simulink model "ALL_JP360_DBW_V6_5_1103"  (R2022a)
settings: Solver=FixedStepAuto  StartTime=0.0  StopTime=inf  FixedStep=0.01  RelTol=1e-3  EnableMultiTasking=on
model workspace (MAT data in the model file):
  g = 9.8
undefined symbols (not defined in the file or in its folder): canChannel, delta_v_p, IPM_Line_C0, IPM_Line_C1, IPM_Line_C2, IPM_Line_C3, M, M_p, MRR_ObjDistX, MRR_ObjDistY, MRR_ObjFusionCamID, MRR_ObjFusionSig, MRR_ObjID, MRR_ObjRelVelX, MRR_ObjRelVelY, MRR_ObjType, MRR_ObjUpdFlg, none, obj_vaild, untracktime, V, videoinput
libraries: canfdmsglib x230, canfdlib x76, slpidlib x24, simulink x18, dspstat3 x14, ctrlSharedLib x1, simulink_extras x1, imaqlib x1, realtime_pacer_lib x1, dspvision x1, visionsinks x1
(part 13 of 55)

== system ALL_JP360_DBW_V6_5_1103/MsgFromCAN/CCAN_GW_MsgFromCAN/CCAN_GW_ESP_Advanced_0x234 ==
  CCAN_GW_ESP_Advanced_0x234FromInData : Inport  OutDataTypeStr=Bus:CAN_FD_MESSAGE_BUS
  Bus Creator : BusCreator  Inputs=24  OutDataTypeStr=Bus:CCAN_GW_ESP_Advanced_0x234  NonVirtualBus=on
  CAN FD Unpack : canfdmsglib/CAN FD Unpack  CANdbFile=HiFire_JPT360_CCAN_Matrix_CAN_V1.72_VP_ADCU.dbc  MsgList=(none)  MsgName=ESP_Advanced_0x234  ProtocolMode=CAN FD  MsgIDType=Standard (11-bit identifier)  MsgIdentifier=564  MsgLength=8  SignalInfo={'Checksum_0x234','56','8','BE','unsigned','Standard','0','1','0','0','255';'ESP_ABAactive','22','1','BE','unsigned','Standard','0','1','0','0','1';'ESP_ABAavailable','21','1','BE','unsigned','Standard','0','1','0','0','1';'ESP_AEBdecActive','18','1','BE','unsigned','Standard','0','1','0','0','1';'ESP_AEBdecAvailable','17','1','BE','unsigned','Standard','0','1','0','0','1';'ESP_AWBactive','26','1','BE','unsigned','Standard','0','1','0','0','1';'ESP_AWBavailable','25','1','BE','unsigned','Standard','0','1','0','0','1';'ESP_BrkFricTqTotAtWhl','40','14','BE','unsigned','Standard','0','1','0','0','10230';'ESP_BrkFricTqTotAtWhlvaild','16','1','BE','unsigned','Standard','0','1','0','0','1';'ESP_CDDActive','8','1','BE','unsigned','Standard','0','1','0','0','1';'ESP_CDDAvailable','23','1','BE','unsigned','Standard','0','1','0','0','1';'ESP_CDD_APAactive','9','1','BE','unsigned','Standard','0','1','0','0','1';'ESP_CDDerror','39','1','BE','unsigned','Standard','0','1','0','0','1';'ESP_DTCactive','24','1','BE','unsigned','Standard','0','1','0','0','1';'ESP_EBDActive','1','1','BE','unsigned','Standard','0','1','0','0','1';'ESP_ECDTempOff','14','1','BE','unsigned','Standard','0','1','0','0','1';'ESP_HBBActive','54','1','BE','unsigned','Standard','0','1','0','0','1';'ESP_NoBrakeForce','15','1','BE','unsigned','Standard','0','1','0','0','1';'ESP_PrefillActive','20','1','BE','unsigned','Standard','0','1','0','0','1';'ESP_PrefillAvailable','19','1','BE','unsigned','Standard','0','1','0','0','1';'ESP_VAMActive','55','1','BE','unsigned','Standard','0','1','0','0','1';'ESP_VDCActive','0','1','BE','unsigned','Standard','0','1','0','0','1';'ESP_VLCerror','38','1','BE','unsigned','Standard','0','1','0','0','1';'RollingCounter_0x234','48','4','BE','unsigned','Standard','0','1','0','0','15'}  IDPort=off  TimestampPort=off  ErrorPort=off  RemotePort=off  LengthPort=off  StatusPort=off  BRSPort=off  ESIPort=off  DLCPort=off  ApplyMinMax=off
      settings: SourceProductBaseCode=XP,ME,VN  DataFormat=CANdb specified signals
  Data Type Conversion1 : DataTypeConversion  OutDataTypeStr=uint8  SaturateOnIntegerOverflow=off  RndMeth=Floor
  Data Type Conversion{2..7,9..23} (21 alike) : DataTypeConversion  OutDataTypeStr=boolean  SaturateOnIntegerOverflow=off  RndMeth=Floor
  Data Type Conversion24 : DataTypeConversion  OutDataTypeStr=int8  SaturateOnIntegerOverflow=off  RndMeth=Floor
  Data Type Conversion8 : DataTypeConversion  OutDataTypeStr=int16  SaturateOnIntegerOverflow=off  RndMeth=Floor
  CCAN_GW_ESP_Advanced_0x234FromOutData : Outport  OutDataTypeStr=Bus:CCAN_GW_ESP_Advanced_0x234
  wires:
  CAN FD Unpack/1 -> Data Type Conversion1/1
  CAN FD Unpack/2 -> Data Type Conversion2/1
  CAN FD Unpack/3 -> Data Type Conversion3/1
  CAN FD Unpack/4 -> Data Type Conversion4/1
  CAN FD Unpack/5 -> Data Type Conversion5/1
  CAN FD Unpack/6 -> Data Type Conversion6/1
  CAN FD Unpack/7 -> Data Type Conversion7/1
  CAN FD Unpack/8 -> Data Type Conversion8/1
  CAN FD Unpack/9 -> Data Type Conversion9/1
  CAN FD Unpack/10 -> Data Type Conversion10/1
  CAN FD Unpack/11 -> Data Type Conversion11/1
  CAN FD Unpack/12 -> Data Type Conversion12/1
  CAN FD Unpack/13 -> Data Type Conversion13/1
  CAN FD Unpack/14 -> Data Type Conversion14/1
  CAN FD Unpack/15 -> Data Type Conversion15/1
  CAN FD Unpack/16 -> Data Type Conversion16/1
  CAN FD Unpack/17 -> Data Type Conversion17/1
  CAN FD Unpack/18 -> Data Type Conversion18/1
  CAN FD Unpack/19 -> Data Type Conversion19/1
  CAN FD Unpack/20 -> Data Type Conversion20/1
  CAN FD Unpack/21 -> Data Type Conversion21/1
  CAN FD Unpack/22 -> Data Type Conversion22/1
  CAN FD Unpack/23 -> Data Type Conversion23/1
  CAN FD Unpack/24 -> Data Type Conversion24/1
  Data Type Conversion1/1 -> Bus Creator/1  "Checksum_0x234"
  Data Type Conversion2/1 -> Bus Creator/2  "ESP_ABAactive"
  Data Type Conversion3/1 -> Bus Creator/3  "ESP_ABAavailable"
  Data Type Conversion4/1 -> Bus Creator/4  "ESP_AEBdecActive"
  Data Type Conversion5/1 -> Bus Creator/5  "ESP_AEBdecAvailable"
  Data Type Conversion6/1 -> Bus Creator/6  "ESP_AWBactive"
  Data Type Conversion7/1 -> Bus Creator/7  "ESP_AWBavailable"
  Data Type Conversion8/1 -> Bus Creator/8  "ESP_BrkFricTqTotAtWhl"
  Data Type Conversion9/1 -> Bus Creator/9  "ESP_BrkFricTqTotAtWhlvaild"
  Data Type Conversion10/1 -> Bus Creator/10  "ESP_CDDActive"
  Data Type Conversion11/1 -> Bus Creator/11  "ESP_CDDAvailable"
  Data Type Conversion12/1 -> Bus Creator/12  "ESP_CDD_APAactive"
  Data Type Conversion13/1 -> Bus Creator/13  "ESP_CDDerror"
  Data Type Conversion14/1 -> Bus Creator/14  "ESP_DTCactive"
  Data Type Conversion15/1 -> Bus Creator/15  "ESP_EBDActive"
  Data Type Conversion16/1 -> Bus Creator/16  "ESP_ECDTempOff"
  Data Type Conversion17/1 -> Bus Creator/17  "ESP_HBBActive"
  Data Type Conversion18/1 -> Bus Creator/18  "ESP_NoBrakeForce"
  Data Type Conversion19/1 -> Bus Creator/19  "ESP_PrefillActive"
  Data Type Conversion20/1 -> Bus Creator/20  "ESP_PrefillAvailable"
  Data Type Conversion21/1 -> Bus Creator/21  "ESP_VAMActive"
  Data Type Conversion22/1 -> Bus Creator/22  "ESP_VDCActive"
  Data Type Conversion23/1 -> Bus Creator/23  "ESP_VLCerror"
  Data Type Conversion24/1 -> Bus Creator/24  "RollingCounter_0x234"
  Bus Creator/1 -> CCAN_GW_ESP_Advanced_0x234FromOutData/1  "CCAN_GW_ESP_Advanced_0x234FromOutData"
  CCAN_GW_ESP_Advanced_0x234FromInData/1 -> CAN FD Unpack/1  "CCAN_GW_ESP_Advanced_0x234FromInData"

== system ALL_JP360_DBW_V6_5_1103/MsgFromCAN/CCAN_GW_MsgFromCAN/CCAN_GW_ESP_AxAy_0x242 ==
  CCAN_GW_ESP_AxAy_0x242FromInData : Inport  OutDataTypeStr=Bus:CAN_FD_MESSAGE_BUS
  Bus Creator : BusCreator  Inputs=8  OutDataTypeStr=Bus:CCAN_GW_ESP_AxAy_0x242  NonVirtualBus=on
  CAN FD Unpack : canfdmsglib/CAN FD Unpack  CANdbFile=HiFire_JPT360_CCAN_Matrix_CAN_V1.72_VP_ADCU.dbc  MsgList=(none)  MsgName=ESP_AxAy_0x242  ProtocolMode=CAN FD  MsgIDType=Standard (11-bit identifier)  MsgIdentifier=578  MsgLength=8  SignalInfo={'Checksum_0x242','56','8','BE','unsigned','Standard','0','1','0','0','255';'ESP_Alat','16','12','BE','unsigned','Standard','0','0.027127','-21.5931','-21.5931','21.5931';'ESP_AlatStatus','54','1','BE','unsigned','Standard','0','1','0','0','1';'ESP_Algt','12','12','BE','unsigned','Standard','0','0.027127','-21.5931','-21.5931','21.5931';'ESP_AlgtStatus','55','1','BE','unsigned','Standard','0','1','0','0','1';'ESP_YawRate','36','12','BE','unsigned','Standard','0','0.001745','-2.0942','-2.0942','5.0498';'ESP_YawRateStatus','53','1','BE','unsigned','Standard','0','1','0','0','1';'RollingCounter_0x242','48','4','BE','unsigned','Standard','0','1','0','0','15'}  IDPort=off  TimestampPort=off  ErrorPort=off  RemotePort=off  LengthPort=off  StatusPort=off  BRSPort=off  ESIPort=off  DLCPort=off  ApplyMinMax=off
      settings: SourceProductBaseCode=XP,ME,VN  DataFormat=CANdb specified signals
  Data Type Conversion1 : DataTypeConversion  OutDataTypeStr=uint8  SaturateOnIntegerOverflow=off  RndMeth=Floor
  Data Type Conversion2 : DataTypeConversion  OutDataTypeStr=single  SaturateOnIntegerOverflow=off  RndMeth=Floor
  Data Type Conversion3 : DataTypeConversion  OutDataTypeStr=boolean  SaturateOnIntegerOverflow=off  RndMeth=Floor
  Data Type Conversion4 : DataTypeConversion  OutDataTypeStr=single  SaturateOnIntegerOverflow=off  RndMeth=Floor
  Data Type Conversion5 : DataTypeConversion  OutDataTypeStr=boolean  SaturateOnIntegerOverflow=off  RndMeth=Floor
  Data Type Conversion6 : DataTypeConversion  OutDataTypeStr=single  SaturateOnIntegerOverflow=off  RndMeth=Floor
  Data Type Conversion7 : DataTypeConversion  OutDataTypeStr=boolean  SaturateOnIntegerOverflow=off  RndMeth=Floor
  Data Type Conversion8 : DataTypeConversion  OutDataTypeStr=int8  SaturateOnIntegerOverflow=off  RndMeth=Floor
  CCAN_GW_ESP_AxAy_0x242FromOutData : Outport  OutDataTypeStr=Bus:CCAN_GW_ESP_AxAy_0x242
  wires:
  CAN FD Unpack/1 -> Data Type Conversion1/1
  CAN FD Unpack/2 -> Data Type Conversion2/1
  CAN FD Unpack/3 -> Data Type Conversion3/1
  CAN FD Unpack/4 -> Data Type Conversion4/1
  CAN FD Unpack/5 -> Data Type Conversion5/1
  CAN FD Unpack/6 -> Data Type Conversion6/1
  CAN FD Unpack/7 -> Data Type Conversion7/1
  CAN FD Unpack/8 -> Data Type Conversion8/1
  Data Type Conversion1/1 -> Bus Creator/1  "Checksum_0x242"
  Data Type Conversion2/1 -> Bus Creator/2  "ESP_Alat"
  Data Type Conversion3/1 -> Bus Creator/3  "ESP_AlatStatus"
  Data Type Conversion4/1 -> Bus Creator/4  "ESP_Algt"
  Data Type Conversion5/1 -> Bus Creator/5  "ESP_AlgtStatus"
  Data Type Conversion6/1 -> Bus Creator/6  "ESP_YawRate"
  Data Type Conversion7/1 -> Bus Creator/7  "ESP_YawRateStatus"
  Data Type Conversion8/1 -> Bus Creator/8  "RollingCounter_0x242"
  Bus Creator/1 -> CCAN_GW_ESP_AxAy_0x242FromOutData/1  "CCAN_GW_ESP_AxAy_0x242FromOutData"
  CCAN_GW_ESP_AxAy_0x242FromInData/1 -> CAN FD Unpack/1  "CCAN_GW_ESP_AxAy_0x242FromInData"

== system ALL_JP360_DBW_V6_5_1103/MsgFromCAN/CCAN_GW_MsgFromCAN/CCAN_GW_ESP_Direction_0x235 ==
  CCAN_GW_ESP_Direction_0x235FromInData : Inport  OutDataTypeStr=Bus:CAN_FD_MESSAGE_BUS
  Bus Creator : BusCreator  Inputs=15  OutDataTypeStr=Bus:CCAN_GW_ESP_Direction_0x235  NonVirtualBus=on
  CAN FD Unpack : canfdmsglib/CAN FD Unpack  CANdbFile=HiFire_JPT360_CCAN_Matrix_CAN_V1.72_VP_ADCU.dbc  MsgList=(none)  MsgName=ESP_Direction_0x235  ProtocolMode=CAN FD  MsgIDType=Standard (11-bit identifier)  MsgIdentifier=565  MsgLength=8  SignalInfo={'Checksum_0x235','56','8','BE','unsigned','Standard','0','1','0','0','255';'ESP_FLWheelDriveDirStatus','33','1','BE','unsigned','Standard','0','1','0','0','1';'ESP_FLWheelDriveDirection','46','2','BE','unsigned','Standard','0','1','0','0','3';'ESP_FRWheelDriveDirStatus','32','1','BE','unsigned','Standard','0','1','0','0','1';'ESP_FRWheelDriveDirection','44','2','BE','unsigned','Standard','0','1','0','0','3';'ESP_RLWheelDriveDirStatus','35','1','BE','unsigned','Standard','0','1','0','0','1';'ESP_RLWheelDriveDirection','42','2','BE','unsigned','Standard','0','1','0','0','3';'ESP_RRWheelDriveDirStatus','34','1','BE','unsigned','Standard','0','1','0','0','1';'ESP_RRWheelDriveDirection','40','2','BE','unsigned','Standard','0','1','0','0','3';'ESP_VehicleStandstill','54','2','BE','unsigned','Standard','0','1','0','0','3';'ESP_WhlMilgReaRLeStatus','52','1','BE','unsigned','Standard','0','1','0','0','1';'ESP_WhlMilgReaRRiStatus','53','1','BE','unsigned','Standard','0','1','0','0','1';'ESP_WhlMilgRearLe','8','16','BE','unsigned','Standard','0','1','0','0','65535';'ESP_WhlMilgRearRe','24','16','BE','unsigned','Standard','0','1','0','0','65535';'RollingCounter_0x235','48','4','BE','unsigned','Standard','0','1','0','0','15'}  IDPort=off  TimestampPort=off  ErrorPort=off  RemotePort=off  LengthPort=off  StatusPort=off  BRSPort=off  ESIPort=off  DLCPort=off  ApplyMinMax=off
      settings: SourceProductBaseCode=XP,ME,VN  DataFormat=CANdb specified signals
  Data Type Conversion1 : DataTypeConversion  OutDataTypeStr=uint8  SaturateOnIntegerOverflow=off  RndMeth=Floor
  Data Type Conversion{3,5,7,9..10,15} (6 alike) : DataTypeConversion  OutDataTypeStr=int8  SaturateOnIntegerOverflow=off  RndMeth=Floor
  Data Type Conversion{2,4,6,8,11..12} (6 alike) : DataTypeConversion  OutDataTypeStr=boolean  SaturateOnIntegerOverflow=off  RndMeth=Floor
  Data Type Conversion13 : DataTypeConversion  OutDataTypeStr=uint16  SaturateOnIntegerOverflow=off  RndMeth=Floor
  Data Type Conversion14 : DataTypeConversion  OutDataTypeStr=uint16  SaturateOnIntegerOverflow=off  RndMeth=Floor
  CCAN_GW_ESP_Direction_0x235FromOutData : Outport  OutDataTypeStr=Bus:CCAN_GW_ESP_Direction_0x235
  wires:
  CAN FD Unpack/1 -> Data Type Conversion1/1
  CAN FD Unpack/2 -> Data Type Conversion2/1
  CAN FD Unpack/3 -> Data Type Conversion3/1
  CAN FD Unpack/4 -> Data Type Conversion4/1
  CAN FD Unpack/5 -> Data Type Conversion5/1
  CAN FD Unpack/6 -> Data Type Conversion6/1
  CAN FD Unpack/7 -> Data Type Conversion7/1
  CAN FD Unpack/8 -> Data Type Conversion8/1
  CAN FD Unpack/9 -> Data Type Conversion9/1
  CAN FD Unpack/10 -> Data Type Conversion10/1
  CAN FD Unpack/11 -> Data Type Conversion11/1
  CAN FD Unpack/12 -> Data Type Conversion12/1
  CAN FD Unpack/13 -> Data Type Conversion13/1
  CAN FD Unpack/14 -> Data Type Conversion14/1
  CAN FD Unpack/15 -> Data Type Conversion15/1
  Data Type Conversion1/1 -> Bus Creator/1  "Checksum_0x235"
  Data Type Conversion2/1 -> Bus Creator/2  "ESP_FLWheelDriveDirStatus"
  Data Type Conversion3/1 -> Bus Creator/3  "ESP_FLWheelDriveDirection"
  Data Type Conversion4/1 -> Bus Creator/4  "ESP_FRWheelDriveDirStatus"
  Data Type Conversion5/1 -> Bus Creator/5  "ESP_FRWheelDriveDirection"
  Data Type Conversion6/1 -> Bus Creator/6  "ESP_RLWheelDriveDirStatus"
  Data Type Conversion7/1 -> Bus Creator/7  "ESP_RLWheelDriveDirection"
  Data Type Conversion8/1 -> Bus Creator/8  "ESP_RRWheelDriveDirStatus"
  Data Type Conversion9/1 -> Bus Creator/9  "ESP_RRWheelDriveDirection"
  Data Type Conversion10/1 -> Bus Creator/10  "ESP_VehicleStandstill"
  Data Type Conversion11/1 -> Bus Creator/11  "ESP_WhlMilgReaRLeStatus"
  Data Type Conversion12/1 -> Bus Creator/12  "ESP_WhlMilgReaRRiStatus"
  Data Type Conversion13/1 -> Bus Creator/13  "ESP_WhlMilgRearLe"
  Data Type Conversion14/1 -> Bus Creator/14  "ESP_WhlMilgRearRe"
  Data Type Conversion15/1 -> Bus Creator/15  "RollingCounter_0x235"
  Bus Creator/1 -> CCAN_GW_ESP_Direction_0x235FromOutData/1  "CCAN_GW_ESP_Direction_0x235FromOutData"
  CCAN_GW_ESP_Direction_0x235FromInData/1 -> CAN FD Unpack/1  "CCAN_GW_ESP_Direction_0x235FromInData"

== system ALL_JP360_DBW_V6_5_1103/MsgFromCAN/CCAN_GW_MsgFromCAN/CCAN_GW_ESP_OBD_Diag_0x600 ==
  CCAN_GW_ESP_OBD_Diag_0x600FromInData : Inport  OutDataTypeStr=Bus:CAN_FD_MESSAGE_BUS
  Bus Creator : BusCreator  Inputs=24  OutDataTypeStr=Bus:CCAN_GW_ESP_OBD_Diag_0x600  NonVirtualBus=on
  CAN FD Unpack : canfdmsglib/CAN FD Unpack  CANdbFile=HiFire_JPT360_CCAN_Matrix_CAN_V1.72_VP_ADCU.dbc  MsgList=(none)  MsgName=ESP_OBD_Diag_0x600  ProtocolMode=CAN FD  MsgIDType=Standard (11-bit identifier)  MsgIdentifier=1536  MsgLength=8  SignalInfo={'Checksum_0x600','56','8','BE','unsigned','Standard','0','1','0','0','255';'ESP_FLWheelSpdSensorFailure','0','1','BE','unsigned','Standard','0','1','0','0','1';'ESP_FLWheelSpdSensorSigFailure','4','1','BE','unsigned','Standard','0','1','0','0','1';'ESP_FLWheelSpdSensor_GND','1','1','BE','unsigned','Standard','0','1','0','0','1';'ESP_FLWheelSpdSensor_Open','3','1','BE','unsigned','Standard','0','1','0','0','1';'ESP_FLWheelSpdSensor_ShtBAT','2','1','BE','unsigned','Standard','0','1','0','0','1';'ESP_FRWheelSpdSensorFailure','5','1','BE','unsigned','Standard','0','1','0','0','1';'ESP_FRWheelSpdSensorSigFailure','9','1','BE','unsigned','Standard','0','1','0','0','1';'ESP_FRWheelSpdSensor_GND','6','1','BE','unsigned','Standard','0','1','0','0','1';'ESP_FRWheelSpdSensor_Open','8','1','BE','unsigned','Standard','0','1','0','0','1';'ESP_FRWheelSpdSensor_ShtBAT','7','1','BE','unsigned','Standard','0','1','0','0','1';'ESP_RLWheelSpdSensorFailure','10','1','BE','unsigned','Standard','0','1','0','0','1';'ESP_RLWheelSpdSensorSigFailure','14','1','BE','unsigned','Standard','0','1','0','0','1';'ESP_RLWheelSpdSensor_GND','11','1','BE','unsigned','Standard','0','1','0','0','1';'ESP_RLWheelSpdSensor_Open','13','1','BE','unsigned','Standard','0','1','0','0','1';'ESP_RLWheelSpdSensor_ShtBAT','12','1','BE','unsigned','Standard','0','1','0','0','1';'ESP_RRWheelSpdSensorFailure','15','1','BE','unsigned','Standard','0','1','0','0','1';'ESP_RRWheelSpdSensorSigFailure','19','1','BE','unsigned','Standard','0','1','0','0','1';'ESP_RRWheelSpdSensor_GND','16','1','BE','unsigned','Standard','0','1','0','0','1';'ESP_RRWheelSpdSensor_Open','18','1','BE','unsigned','Standard','0','1','0','0','1';'ESP_RRWheelSpdSensor_ShtBAT','17','1','BE','unsigned','Standard','0','1','0','0','1';'ESP_WheelSpdSensorEcuError','21','1','BE','unsigned','Standard','0','1','0','0','1';'ESP_WheelSpdSensorError','20','1','BE','unsigned','Standard','0','1','0','0','1';'Rolling_counter_0x600','48','4','BE','unsigned','Standard','0','1','0','0','15'}  IDPort=off  TimestampPort=off  ErrorPort=off  RemotePort=off  LengthPort=off  StatusPort=off  BRSPort=off  ESIPort=off  DLCPort=off  ApplyMinMax=off
      settings: SourceProductBaseCode=XP,ME,VN  DataFormat=CANdb specified signals
  Data Type Conversion1 : DataTypeConversion  OutDataTypeStr=uint8  SaturateOnIntegerOverflow=off  RndMeth=Floor
  Data Type Conversion{2..23} (22 alike) : DataTypeConversion  OutDataTypeStr=boolean  SaturateOnIntegerOverflow=off  RndMeth=Floor
  Data Type Conversion24 : DataTypeConversion  OutDataTypeStr=int8  SaturateOnIntegerOverflow=off  RndMeth=Floor
  CCAN_GW_ESP_OBD_Diag_0x600FromOutData : Outport  OutDataTypeStr=Bus:CCAN_GW_ESP_OBD_Diag_0x600
  wires:
  CAN FD Unpack/1 -> Data Type Conversion1/1
  CAN FD Unpack/2 -> Data Type Conversion2/1
  CAN FD Unpack/3 -> Data Type Conversion3/1
  CAN FD Unpack/4 -> Data Type Conversion4/1
  CAN FD Unpack/5 -> Data Type Conversion5/1
  CAN FD Unpack/6 -> Data Type Conversion6/1
  CAN FD Unpack/7 -> Data Type Conversion7/1
  CAN FD Unpack/8 -> Data Type Conversion8/1
  CAN FD Unpack/9 -> Data Type Conversion9/1
  CAN FD Unpack/10 -> Data Type Conversion10/1
  CAN FD Unpack/11 -> Data Type Conversion11/1
  CAN FD Unpack/12 -> Data Type Conversion12/1
  CAN FD Unpack/13 -> Data Type Conversion13/1
  CAN FD Unpack/14 -> Data Type Conversion14/1
  CAN FD Unpack/15 -> Data Type Conversion15/1
  CAN FD Unpack/16 -> Data Type Conversion16/1
  CAN FD Unpack/17 -> Data Type Conversion17/1
  CAN FD Unpack/18 -> Data Type Conversion18/1
  CAN FD Unpack/19 -> Data Type Conversion19/1
  CAN FD Unpack/20 -> Data Type Conversion20/1
  CAN FD Unpack/21 -> Data Type Conversion21/1
  CAN FD Unpack/22 -> Data Type Conversion22/1
  CAN FD Unpack/23 -> Data Type Conversion23/1
  CAN FD Unpack/24 -> Data Type Conversion24/1
  Data Type Conversion1/1 -> Bus Creator/1  "Checksum_0x600"
  Data Type Conversion2/1 -> Bus Creator/2  "ESP_FLWheelSpdSensorFailure"
  Data Type Conversion3/1 -> Bus Creator/3  "ESP_FLWheelSpdSensorSigFailure"
  Data Type Conversion4/1 -> Bus Creator/4  "ESP_FLWheelSpdSensor_GND"
  Data Type Conversion5/1 -> Bus Creator/5  "ESP_FLWheelSpdSensor_Open"
  Data Type Conversion6/1 -> Bus Creator/6  "ESP_FLWheelSpdSensor_ShtBAT"
  Data Type Conversion7/1 -> Bus Creator/7  "ESP_FRWheelSpdSensorFailure"
  Data Type Conversion8/1 -> Bus Creator/8  "ESP_FRWheelSpdSensorSigFailure"
  Data Type Conversion9/1 -> Bus Creator/9  "ESP_FRWheelSpdSensor_GND"
  Data Type Conversion10/1 -> Bus Creator/10  "ESP_FRWheelSpdSensor_Open"
  Data Type Conversion11/1 -> Bus Creator/11  "ESP_FRWheelSpdSensor_ShtBAT"
  Data Type Conversion12/1 -> Bus Creator/12  "ESP_RLWheelSpdSensorFailure"
  Data Type Conversion13/1 -> Bus Creator/13  "ESP_RLWheelSpdSensorSigFailure"
  Data Type Conversion14/1 -> Bus Creator/14  "ESP_RLWheelSpdSensor_GND"
  Data Type Conversion15/1 -> Bus Creator/15  "ESP_RLWheelSpdSensor_Open"
  Data Type Conversion16/1 -> Bus Creator/16  "ESP_RLWheelSpdSensor_ShtBAT"
  Data Type Conversion17/1 -> Bus Creator/17  "ESP_RRWheelSpdSensorFailure"
  Data Type Conversion18/1 -> Bus Creator/18  "ESP_RRWheelSpdSensorSigFailure"
  Data Type Conversion19/1 -> Bus Creator/19  "ESP_RRWheelSpdSensor_GND"
  Data Type Conversion20/1 -> Bus Creator/20  "ESP_RRWheelSpdSensor_Open"
  Data Type Conversion21/1 -> Bus Creator/21  "ESP_RRWheelSpdSensor_ShtBAT"
  Data Type Conversion22/1 -> Bus Creator/22  "ESP_WheelSpdSensorEcuError"
  Data Type Conversion23/1 -> Bus Creator/23  "ESP_WheelSpdSensorError"
  Data Type Conversion24/1 -> Bus Creator/24  "Rolling_counter_0x600"
  Bus Creator/1 -> CCAN_GW_ESP_OBD_Diag_0x600FromOutData/1  "CCAN_GW_ESP_OBD_Diag_0x600FromOutData"
  CCAN_GW_ESP_OBD_Diag_0x600FromInData/1 -> CAN FD Unpack/1  "CCAN_GW_ESP_OBD_Diag_0x600FromInData"

== system ALL_JP360_DBW_V6_5_1103/MsgFromCAN/CCAN_GW_MsgFromCAN/CCAN_GW_ESP_Pressure_0x241 ==
  CCAN_GW_ESP_Pressure_0x241FromInData : Inport  OutDataTypeStr=Bus:CAN_FD_MESSAGE_BUS
  Bus Creator : BusCreator  Inputs=11  OutDataTypeStr=Bus:CCAN_GW_ESP_Pressure_0x241  NonVirtualBus=on
  CAN FD Unpack : canfdmsglib/CAN FD Unpack  CANdbFile=HiFire_JPT360_CCAN_Matrix_CAN_V1.72_VP_ADCU.dbc  MsgList=(none)  MsgName=ESP_Pressure_0x241  ProtocolMode=CAN FD  MsgIDType=Standard (11-bit identifier)  MsgIdentifier=577  MsgLength=8  SignalInfo={'ABS_ForbidRegen_Active','54','1','BE','unsigned','Standard','0','1','0','0','1';'Checksum_0x241','56','8','BE','unsigned','Standard','0','1','0','0','255';'ESP_Master_Cylinder_Pressure','12','12','BE','unsigned','Standard','0','0.0625','0','0','255.9375';'ESP_Master_Cylinder_Pressure_Status','55','1','BE','unsigned','Standard','0','1','0','0','1';'ESP_MbRegenTargetWhl','32','16','BE','unsigned','Standard','0','1','-30000','-30000','30000';'ESP_MbRegenTargetWhlQualifier','52','2','BE','unsigned','Standard','0','1','0','0','2';'ESP_PresOffsetMasterCylinder','43','5','BE','unsigned','Standard','0','1','-15','-15','15';'ESP_PresOffsetMasterCylinderValid','42','1','BE','unsigned','Standard','0','1','0','0','1';'ESP_TrfCaseModReqdByEsp','40','2','BE','unsigned','Standard','0','1','0','0','3';'ESP_TrfCaseTqLmtdByEsp','16','12','BE','unsigned','Standard','0','1','0','0','4095';'RollingCounter_0x241','48','4','BE','unsigned','Standard','0','1','0','0','15'}  IDPort=off  TimestampPort=off  ErrorPort=off  RemotePort=off  LengthPort=off  StatusPort=off  BRSPort=off  ESIPort=off  DLCPort=off  ApplyMinMax=off
      settings: SourceProductBaseCode=XP,ME,VN  DataFormat=CANdb specified signals
  Data Type Conversion1 : DataTypeConversion  OutDataTypeStr=boolean  SaturateOnIntegerOverflow=off  RndMeth=Floor
  Data Type Conversion10 : DataTypeConversion  OutDataTypeStr=int16  SaturateOnIntegerOverflow=off  RndMeth=Floor
  Data Type Conversion{6..7,9,11} (4 alike) : DataTypeConversion  OutDataTypeStr=int8  SaturateOnIntegerOverflow=off  RndMeth=Floor
  Data Type Conversion2 : DataTypeConversion  OutDataTypeStr=uint8  SaturateOnIntegerOverflow=off  RndMeth=Floor
  Data Type Conversion3 : DataTypeConversion  OutDataTypeStr=single  SaturateOnIntegerOverflow=off  RndMeth=Floor
  Data Type Conversion4 : DataTypeConversion  OutDataTypeStr=boolean  SaturateOnIntegerOverflow=off  RndMeth=Floor
  Data Type Conversion5 : DataTypeConversion  OutDataTypeStr=int16  SaturateOnIntegerOverflow=off  RndMeth=Floor
  Data Type Conversion8 : DataTypeConversion  OutDataTypeStr=boolean  SaturateOnIntegerOverflow=off  RndMeth=Floor
  CCAN_GW_ESP_Pressure_0x241FromOutData : Outport  OutDataTypeStr=Bus:CCAN_GW_ESP_Pressure_0x241
  wires:
  CAN FD Unpack/1 -> Data Type Conversion1/1
  CAN FD Unpack/2 -> Data Type Conversion2/1
  CAN FD Unpack/3 -> Data Type Conversion3/1
  CAN FD Unpack/4 -> Data Type Conversion4/1
  CAN FD Unpack/5 -> Data Type Conversion5/1
  CAN FD Unpack/6 -> Data Type Conversion6/1
  CAN FD Unpack/7 -> Data Type Conversion7/1
  CAN FD Unpack/8 -> Data Type Conversion8/1
  CAN FD Unpack/9 -> Data Type Conversion9/1
  CAN FD Unpack/10 -> Data Type Conversion10/1
  CAN FD Unpack/11 -> Data Type Conversion11/1
  Data Type Conversion1/1 -> Bus Creator/1  "ABS_ForbidRegen_Active"
  Data Type Conversion2/1 -> Bus Creator/2  "Checksum_0x241"
  Data Type Conversion3/1 -> Bus Creator/3  "ESP_Master_Cylinder_Pressure"
  Data Type Conversion4/1 -> Bus Creator/4  "ESP_Master_Cylinder_Pressure_Status"
  Data Type Conversion5/1 -> Bus Creator/5  "ESP_MbRegenTargetWhl"
  Data Type Conversion6/1 -> Bus Creator/6  "ESP_MbRegenTargetWhlQualifier"
  Data Type Conversion7/1 -> Bus Creator/7  "ESP_PresOffsetMasterCylinder"
  Data Type Conversion8/1 -> Bus Creator/8  "ESP_PresOffsetMasterCylinderValid"
  Data Type Conversion9/1 -> Bus Creator/9  "ESP_TrfCaseModReqdByEsp"
  Data Type Conversion10/1 -> Bus Creator/10  "ESP_TrfCaseTqLmtdByEsp"
  Data Type Conversion11/1 -> Bus Creator/11  "RollingCounter_0x241"
  Bus Creator/1 -> CCAN_GW_ESP_Pressure_0x241FromOutData/1  "CCAN_GW_ESP_Pressure_0x241FromOutData"
  CCAN_GW_ESP_Pressure_0x241FromInData/1 -> CAN FD Unpack/1  "CCAN_GW_ESP_Pressure_0x241FromInData"

== system ALL_JP360_DBW_V6_5_1103/MsgFromCAN/CCAN_GW_MsgFromCAN/CCAN_GW_ESP_RAW_0x212 ==
  CCAN_GW_ESP_RAW_0x212FromInData : Inport  OutDataTypeStr=Bus:CAN_FD_MESSAGE_BUS
  Bus Creator : BusCreator  Inputs=10  OutDataTypeStr=Bus:CCAN_GW_ESP_RAW_0x212  NonVirtualBus=on
  CAN FD Unpack : canfdmsglib/CAN FD Unpack  CANdbFile=HiFire_JPT360_CCAN_Matrix_CAN_V1.72_VP_ADCU.dbc  MsgList=(none)  MsgName=ESP_RAW_0x212  ProtocolMode=CAN FD  MsgIDType=Standard (11-bit identifier)  MsgIdentifier=530  MsgLength=8  SignalInfo={'Checksum_0x212','56','8','BE','unsigned','Standard','0','1','0','0','255';'ESP_vxwWheelFLValid','55','1','BE','unsigned','Standard','0','1','0','0','1';'ESP_vxwWheelFRValid','54','1','BE','unsigned','Standard','0','1','0','0','1';'ESP_vxwWheelRLValid','53','1','BE','unsigned','Standard','0','1','0','0','1';'ESP_vxwWheelRRValid','52','1','BE','unsigned','Standard','0','1','0','0','1';'ESP_vxwWheelRawFL','12','12','BE','unsigned','Standard','0','0.05625','0','0','230.2875';'ESP_vxwWheelRawFR','16','12','BE','unsigned','Standard','0','0.05625','0','0','230.2875';'ESP_vxwWheelRawRL','36','12','BE','unsigned','Standard','0','0.05625','0','0','230.2875';'ESP_vxwWheelRawRR','40','12','BE','unsigned','Standard','0','0.05625','0','0','230.2875';'RollingCounter_0x212','48','4','BE','unsigned','Standard','0','1','0','0','15'}  IDPort=off  TimestampPort=off  ErrorPort=off  RemotePort=off  LengthPort=off  StatusPort=off  BRSPort=off  ESIPort=off  DLCPort=off  ApplyMinMax=off
      settings: SourceProductBaseCode=XP,ME,VN  DataFormat=CANdb specified signals
  Data Type Conversion1 : DataTypeConversion  OutDataTypeStr=uint8  SaturateOnIntegerOverflow=off  RndMeth=Floor
  Data Type Conversion10 : DataTypeConversion  OutDataTypeStr=int8  SaturateOnIntegerOverflow=off  RndMeth=Floor
  Data Type Conversion{2..5} (4 alike) : DataTypeConversion  OutDataTypeStr=boolean  SaturateOnIntegerOverflow=off  RndMeth=Floor
  Data Type Conversion{6..9} (4 alike) : DataTypeConversion  OutDataTypeStr=single  SaturateOnIntegerOverflow=off  RndMeth=Floor
  CCAN_GW_ESP_RAW_0x212FromOutData : Outport  OutDataTypeStr=Bus:CCAN_GW_ESP_RAW_0x212
  wires:
  CAN FD Unpack/1 -> Data Type Conversion1/1
  CAN FD Unpack/2 -> Data Type Conversion2/1
  CAN FD Unpack/3 -> Data Type Conversion3/1
  CAN FD Unpack/4 -> Data Type Conversion4/1
  CAN FD Unpack/5 -> Data Type Conversion5/1
  CAN FD Unpack/6 -> Data Type Conversion6/1
  CAN FD Unpack/7 -> Data Type Conversion7/1
  CAN FD Unpack/8 -> Data Type Conversion8/1
  CAN FD Unpack/9 -> Data Type Conversion9/1
  CAN FD Unpack/10 -> Data Type Conversion10/1
  Data Type Conversion1/1 -> Bus Creator/1  "Checksum_0x212"
  Data Type Conversion2/1 -> Bus Creator/2  "ESP_vxwWheelFLValid"
  Data Type Conversion3/1 -> Bus Creator/3  "ESP_vxwWheelFRValid"
  Data Type Conversion4/1 -> Bus Creator/4  "ESP_vxwWheelRLValid"
  Data Type Conversion5/1 -> Bus Creator/5  "ESP_vxwWheelRRValid"
  Data Type Conversion6/1 -> Bus Creator/6  "ESP_vxwWheelRawFL"
  Data Type Conversion7/1 -> Bus Creator/7  "ESP_vxwWheelRawFR"
  Data Type Conversion8/1 -> Bus Creator/8  "ESP_vxwWheelRawRL"
  Data Type Conversion9/1 -> Bus Creator/9  "ESP_vxwWheelRawRR"
  Data Type Conversion10/1 -> Bus Creator/10  "RollingCounter_0x212"
  Bus Creator/1 -> CCAN_GW_ESP_RAW_0x212FromOutData/1  "CCAN_GW_ESP_RAW_0x212FromOutData"
  CCAN_GW_ESP_RAW_0x212FromInData/1 -> CAN FD Unpack/1  "CCAN_GW_ESP_RAW_0x212FromInData"

== system ALL_JP360_DBW_V6_5_1103/MsgFromCAN/CCAN_GW_MsgFromCAN/CCAN_GW_ESP_RPMF_0x213 ==
  CCAN_GW_ESP_RPMF_0x213FromInData : Inport  OutDataTypeStr=Bus:CAN_FD_MESSAGE_BUS
  Bus Creator : BusCreator  Inputs=10  OutDataTypeStr=Bus:CCAN_GW_ESP_RPMF_0x213  NonVirtualBus=on
  CAN FD Unpack : canfdmsglib/CAN FD Unpack  CANdbFile=HiFire_JPT360_CCAN_Matrix_CAN_V1.72_VP_ADCU.dbc  MsgList=(none)  MsgName=ESP_RPMF_0x213  ProtocolMode=CAN FD  MsgIDType=Standard (11-bit identifier)  MsgIdentifier=531  MsgLength=8  SignalInfo={'Checksum_0x213','56','8','BE','unsigned','Standard','0','1','0','0','255';'ESP_DSTSts','42','2','BE','unsigned','Standard','0','1','0','0','2';'ESP_DSTTrqReq','45','11','BE','unsigned','Standard','0','0.01','-10.24','-10.24','10.22';'ESP_DSTTrqReqValid','44','1','BE','unsigned','Standard','0','1','0','0','1';'ESP_TrailerSMSts','40','2','BE','unsigned','Standard','0','1','0','0','2';'ESP_WheelRpmFL','9','15','BE','unsigned','Standard','0','0.0625','0','0','2047.875';'ESP_WheelRpmFLValid','8','1','BE','unsigned','Standard','0','1','0','0','1';'ESP_WheelRpmFR','25','15','BE','unsigned','Standard','0','0.0625','0','0','2047.875';'ESP_WheelRpmFRValid','24','1','BE','unsigned','Standard','0','1','0','0','1';'RollingCounter_0x213','48','4','BE','unsigned','Standard','0','1','0','0','15'}  IDPort=off  TimestampPort=off  ErrorPort=off  RemotePort=off  LengthPort=off  StatusPort=off  BRSPort=off  ESIPort=off  DLCPort=off  ApplyMinMax=off
      settings: SourceProductBaseCode=XP,ME,VN  DataFormat=CANdb specified signals
  Data Type Conversion1 : DataTypeConversion  OutDataTypeStr=uint8  SaturateOnIntegerOverflow=off  RndMeth=Floor
  Data Type Conversion10 : DataTypeConversion  OutDataTypeStr=int8  SaturateOnIntegerOverflow=off  RndMeth=Floor
  Data Type Conversion2 : DataTypeConversion  OutDataTypeStr=int8  SaturateOnIntegerOverflow=off  RndMeth=Floor
  Data Type Conversion3 : DataTypeConversion  OutDataTypeStr=single  SaturateOnIntegerOverflow=off  RndMeth=Floor
  Data Type Conversion4 : DataTypeConversion  OutDataTypeStr=boolean  SaturateOnIntegerOverflow=off  RndMeth=Floor
  Data Type Conversion5 : DataTypeConversion  OutDataTypeStr=int8  SaturateOnIntegerOverflow=off  RndMeth=Floor
  Data Type Conversion6 : DataTypeConversion  OutDataTypeStr=single  SaturateOnIntegerOverflow=off  RndMeth=Floor
  Data Type Conversion7 : DataTypeConversion  OutDataTypeStr=boolean  SaturateOnIntegerOverflow=off  RndMeth=Floor
  Data Type Conversion8 : DataTypeConversion  OutDataTypeStr=single  SaturateOnIntegerOverflow=off  RndMeth=Floor
  Data Type Conversion9 : DataTypeConversion  OutDataTypeStr=boolean  SaturateOnIntegerOverflow=off  RndMeth=Floor
  CCAN_GW_ESP_RPMF_0x213FromOutData : Outport  OutDataTypeStr=Bus:CCAN_GW_ESP_RPMF_0x213
  wires:
  CAN FD Unpack/1 -> Data Type Conversion1/1
  CAN FD Unpack/2 -> Data Type Conversion2/1
  CAN FD Unpack/3 -> Data Type Conversion3/1
  CAN FD Unpack/4 -> Data Type Conversion4/1
  CAN FD Unpack/5 -> Data Type Conversion5/1
  CAN FD Unpack/6 -> Data Type Conversion6/1
  CAN FD Unpack/7 -> Data Type Conversion7/1
  CAN FD Unpack/8 -> Data Type Conversion8/1
  CAN FD Unpack/9 -> Data Type Conversion9/1
  CAN FD Unpack/10 -> Data Type Conversion10/1
  Data Type Conversion1/1 -> Bus Creator/1  "Checksum_0x213"
  Data Type Conversion2/1 -> Bus Creator/2  "ESP_DSTSts"
  Data Type Conversion3/1 -> Bus Creator/3  "ESP_DSTTrqReq"
  Data Type Conversion4/1 -> Bus Creator/4  "ESP_DSTTrqReqValid"
  Data Type Conversion5/1 -> Bus Creator/5  "ESP_TrailerSMSts"
  Data Type Conversion6/1 -> Bus Creator/6  "ESP_WheelRpmFL"
  Data Type Conversion7/1 -> Bus Creator/7  "ESP_WheelRpmFLValid"
  Data Type Conversion8/1 -> Bus Creator/8  "ESP_WheelRpmFR"
  Data Type Conversion9/1 -> Bus Creator/9  "ESP_WheelRpmFRValid"
  Data Type Conversion10/1 -> Bus Creator/10  "RollingCounter_0x213"
  Bus Creator/1 -> CCAN_GW_ESP_RPMF_0x213FromOutData/1  "CCAN_GW_ESP_RPMF_0x213FromOutData"
  CCAN_GW_ESP_RPMF_0x213FromInData/1 -> CAN FD Unpack/1  "CCAN_GW_ESP_RPMF_0x213FromInData"

== system ALL_JP360_DBW_V6_5_1103/MsgFromCAN/CCAN_GW_MsgFromCAN/CCAN_GW_ESP_RPMR_0x214 ==
  CCAN_GW_ESP_RPMR_0x214FromInData : Inport  OutDataTypeStr=Bus:CAN_FD_MESSAGE_BUS
  Bus Creator : BusCreator  Inputs=6  OutDataTypeStr=Bus:CCAN_GW_ESP_RPMR_0x214  NonVirtualBus=on
  CAN FD Unpack : canfdmsglib/CAN FD Unpack  CANdbFile=HiFire_JPT360_CCAN_Matrix_CAN_V1.72_VP_ADCU.dbc  MsgList=(none)  MsgName=ESP_RPMR_0x214  ProtocolMode=CAN FD  MsgIDType=Standard (11-bit identifier)  MsgIdentifier=532  MsgLength=8  SignalInfo={'Checksum_0x214','56','8','BE','unsigned','Standard','0','1','0','0','255';'ESP_WheelRpmRL','9','15','BE','unsigned','Standard','0','0.0625','0','0','2047.875';'ESP_WheelRpmRLValid','8','1','BE','unsigned','Standard','0','1','0','0','1';'ESP_WheelRpmRR','25','15','BE','unsigned','Standard','0','0.0625','0','0','2047.875';'ESP_WheelRpmRRValid','24','1','BE','unsigned','Standard','0','1','0','0','1';'RollingCounter_0x214','48','4','BE','unsigned','Standard','0','1','0','0','15'}  IDPort=off  TimestampPort=off  ErrorPort=off  RemotePort=off  LengthPort=off  StatusPort=off  BRSPort=off  ESIPort=off  DLCPort=off  ApplyMinMax=off
      settings: SourceProductBaseCode=XP,ME,VN  DataFormat=CANdb specified signals
  Data Type Conversion1 : DataTypeConversion  OutDataTypeStr=uint8  SaturateOnIntegerOverflow=off  RndMeth=Floor
  Data Type Conversion2 : DataTypeConversion  OutDataTypeStr=single  SaturateOnIntegerOverflow=off  RndMeth=Floor
  Data Type Conversion3 : DataTypeConversion  OutDataTypeStr=boolean  SaturateOnIntegerOverflow=off  RndMeth=Floor
  Data Type Conversion4 : DataTypeConversion  OutDataTypeStr=single  SaturateOnIntegerOverflow=off  RndMeth=Floor
  Data Type Conversion5 : DataTypeConversion  OutDataTypeStr=boolean  SaturateOnIntegerOverflow=off  RndMeth=Floor
  Data Type Conversion6 : DataTypeConversion  OutDataTypeStr=int8  SaturateOnIntegerOverflow=off  RndMeth=Floor
  CCAN_GW_ESP_RPMR_0x214FromOutData : Outport  OutDataTypeStr=Bus:CCAN_GW_ESP_RPMR_0x214
  wires:
  CAN FD Unpack/1 -> Data Type Conversion1/1
  CAN FD Unpack/2 -> Data Type Conversion2/1
  CAN FD Unpack/3 -> Data Type Conversion3/1
  CAN FD Unpack/4 -> Data Type Conversion4/1
  CAN FD Unpack/5 -> Data Type Conversion5/1
  CAN FD Unpack/6 -> Data Type Conversion6/1
  Data Type Conversion1/1 -> Bus Creator/1  "Checksum_0x214"
  Data Type Conversion2/1 -> Bus Creator/2  "ESP_WheelRpmRL"
  Data Type Conversion3/1 -> Bus Creator/3  "ESP_WheelRpmRLValid"
  Data Type Conversion4/1 -> Bus Creator/4  "ESP_WheelRpmRR"
  Data Type Conversion5/1 -> Bus Creator/5  "ESP_WheelRpmRRValid"
  Data Type Conversion6/1 -> Bus Creator/6  "RollingCounter_0x214"
  Bus Creator/1 -> CCAN_GW_ESP_RPMR_0x214FromOutData/1  "CCAN_GW_ESP_RPMR_0x214FromOutData"
  CCAN_GW_ESP_RPMR_0x214FromInData/1 -> CAN FD Unpack/1  "CCAN_GW_ESP_RPMR_0x214FromInData"

== system ALL_JP360_DBW_V6_5_1103/MsgFromCAN/CCAN_GW_MsgFromCAN/CCAN_GW_ESP_Status_0x243 ==
  CCAN_GW_ESP_Status_0x243FromInData : Inport  OutDataTypeStr=Bus:CAN_FD_MESSAGE_BUS
  Bus Creator : BusCreator  Inputs=38  OutDataTypeStr=Bus:CCAN_GW_ESP_Status_0x243  NonVirtualBus=on
  CAN FD Unpack : canfdmsglib/CAN FD Unpack  CANdbFile=HiFire_JPT360_CCAN_Matrix_CAN_V1.72_VP_ADCU.dbc  MsgList=(none)  MsgName=ESP_Status_0x243  ProtocolMode=CAN FD  MsgIDType=Standard (11-bit identifier)  MsgIdentifier=579  MsgLength=8  SignalInfo={'ABS_HAZActive','2','1','BE','unsigned','Standard','0','1','0','0','1';'Checksum_0x243','56','8','BE','unsigned','Standard','0','1','0','0','255';'EBS_EbsFlgFlt','43','1','BE','unsigned','Standard','0','1','0','0','1';'ESP_ATS_Driving_mode_confirm','28','4','BE','unsigned','Standard','0','1','0','0','15';'ESP_ATS_Fault_mode','27','1','BE','unsigned','Standard','0','1','0','0','1';'ESP_ATS_failure_Lamp','24','3','BE','unsigned','Standard','0','1','0','0','7';'ESP_AVHWarningMessage','20','1','BE','unsigned','Standard','0','1','0','0','1';'ESP_AvhActive','21','1','BE','unsigned','Standard','0','1','0','0','1';'ESP_AvhAvabliable','23','1','BE','unsigned','Standard','0','1','0','0','1';'ESP_AvhStandby','22','1','BE','unsigned','Standard','0','1','0','0','1';'ESP_CCSwitchOff','8','1','BE','unsigned','Standard','0','1','0','0','1';'ESP_CdpActive','15','1','BE','unsigned','Standard','0','1','0','0','1';'ESP_CdpAvailable','14','1','BE','unsigned','Standard','0','1','0','0','1';'ESP_Driving_mode_req','36','4','BE','unsigned','Standard','0','1','0','0','15';'ESP_EPBErrorStatus','6','2','BE','unsigned','Standard','0','1','0','0','3';'ESP_EPBStatus','3','3','BE','unsigned','Standard','0','1','0','0','7';'ESP_EPBWarningMessage1','19','1','BE','unsigned','Standard','0','1','0','0','1';'ESP_EPBWarningMessage2','18','1','BE','unsigned','Standard','0','1','0','0','1';'ESP_EPBWarningMessage3','17','1','BE','unsigned','Standard','0','1','0','0','1';'ESP_ESPInfoLamp','44','1','BE','unsigned','Standard','0','1','0','0','1';'ESP_EspCtrlActv','35','1','BE','unsigned','Standard','0','1','0','0','1';'ESP_EspEnableSts','45','1','BE','unsigned','Standard','0','1','0','0','1';'ESP_GearShiftPrevn','46','2','BE','unsigned','Standard','0','1','0','0','3';'ESP_HBBActive_NBS','16','1','BE','unsigned','Standard','0','1','0','0','1';'ESP_HBBstatus','54','2','BE','unsigned','Standard','0','1','0','0','2';'ESP_HBCActive_NBS','53','1','BE','unsigned','Standard','0','1','0','0','1';'ESP_HDCActive','11','2','BE','unsigned','Standard','0','1','0','0','2';'ESP_HDCAvailable','9','1','BE','unsigned','Standard','0','1','0','0','1';'ESP_HHCActive','1','1','BE','unsigned','Standard','0','1','0','0','1';'ESP_HHCAvailable','0','1','BE','unsigned','Standard','0','1','0','0','1';'ESP_LdmBLC_BLRequestController','13','1','BE','unsigned','Standard','0','1','0','0','1';'ESP_SCMSts','41','2','BE','unsigned','Standard','0','1','0','0','3';'ESP_TcsCtrlActv','34','1','BE','unsigned','Standard','0','1','0','0','1';'ESP_TcsFlgFlt','33','1','BE','unsigned','Standard','0','1','0','0','1';'ESP_VAMstatus','10','1','BE','unsigned','Standard','0','1','0','0','1';'ESP_VdcFlgFlt','32','1','BE','unsigned','Standard','0','1','0','0','1';'RollerBenchModeSts','52','1','BE','unsigned','Standard','0','1','0','0','1';'RollingCounter_0x243','48','4','BE','unsigned','Standard','0','1','0','0','15'}  IDPort=off  TimestampPort=off  ErrorPort=off  RemotePort=off  LengthPort=off  StatusPort=off  BRSPort=off  ESIPort=off  DLCPort=off  ApplyMinMax=off
      settings: SourceProductBaseCode=XP,ME,VN  DataFormat=CANdb specified signals
  Data Type Conversion{1,3,5,7..13,17..22,24,26,28..31,33..37} (27 alike) : DataTypeConversion  OutDataTypeStr=boolean  SaturateOnIntegerOverflow=off  RndMeth=Floor
  Data Type Conversion{4,6,14..16,23,25,27,32,38} (10 alike) : DataTypeConversion  OutDataTypeStr=int8  SaturateOnIntegerOverflow=off  RndMeth=Floor
  Data Type Conversion2 : DataTypeConversion  OutDataTypeStr=uint8  SaturateOnIntegerOverflow=off  RndMeth=Floor
  CCAN_GW_ESP_Status_0x243FromOutData : Outport  OutDataTypeStr=Bus:CCAN_GW_ESP_Status_0x243
  wires:
  CAN FD Unpack/1 -> Data Type Conversion1/1
  CAN FD Unpack/2 -> Data Type Conversion2/1
  CAN FD Unpack/3 -> Data Type Conversion3/1
  CAN FD Unpack/4 -> Data Type Conversion4/1
  CAN FD Unpack/5 -> Data Type Conversion5/1
  CAN FD Unpack/6 -> Data Type Conversion6/1
  CAN FD Unpack/7 -> Data Type Conversion7/1
  CAN FD Unpack/8 -> Data Type Conversion8/1
  CAN FD Unpack/9 -> Data Type Conversion9/1
  CAN FD Unpack/10 -> Data Type Conversion10/1
  CAN FD Unpack/11 -> Data Type Conversion11/1
  CAN FD Unpack/12 -> Data Type Conversion12/1
  CAN FD Unpack/13 -> Data Type Conversion13/1
  CAN FD Unpack/14 -> Data Type Conversion14/1
  CAN FD Unpack/15 -> Data Type Conversion15/1
  CAN FD Unpack/16 -> Data Type Conversion16/1
  CAN FD Unpack/17 -> Data Type Conversion17/1
  CAN FD Unpack/18 -> Data Type Conversion18/1
  CAN FD Unpack/19 -> Data Type Conversion19/1
  CAN FD Unpack/20 -> Data Type Conversion20/1
  CAN FD Unpack/21 -> Data Type Conversion21/1
  CAN FD Unpack/22 -> Data Type Conversion22/1
  CAN FD Unpack/23 -> Data Type Conversion23/1
  CAN FD Unpack/24 -> Data Type Conversion24/1
  CAN FD Unpack/25 -> Data Type Conversion25/1
  CAN FD Unpack/26 -> Data Type Conversion26/1
  CAN FD Unpack/27 -> Data Type Conversion27/1
  CAN FD Unpack/28 -> Data Type Conversion28/1
  CAN FD Unpack/29 -> Data Type Conversion29/1
  CAN FD Unpack/30 -> Data Type Conversion30/1
  CAN FD Unpack/31 -> Data Type Conversion31/1
  CAN FD Unpack/32 -> Data Type Conversion32/1
  CAN FD Unpack/33 -> Data Type Conversion33/1
  CAN FD Unpack/34 -> Data Type Conversion34/1
  CAN FD Unpack/35 -> Data Type Conversion35/1
  CAN FD Unpack/36 -> Data Type Conversion36/1
  CAN FD Unpack/37 -> Data Type Conversion37/1
  CAN FD Unpack/38 -> Data Type Conversion38/1
  Data Type Conversion1/1 -> Bus Creator/1  "ABS_HAZActive"
  Data Type Conversion2/1 -> Bus Creator/2  "Checksum_0x243"
  Data Type Conversion3/1 -> Bus Creator/3  "EBS_EbsFlgFlt"
  Data Type Conversion4/1 -> Bus Creator/4  "ESP_ATS_Driving_mode_confirm"
  Data Type Conversion5/1 -> Bus Creator/5  "ESP_ATS_Fault_mode"
  Data Type Conversion6/1 -> Bus Creator/6  "ESP_ATS_failure_Lamp"
  Data Type Conversion7/1 -> Bus Creator/7  "ESP_AVHWarningMessage"
  Data Type Conversion8/1 -> Bus Creator/8  "ESP_AvhActive"
  Data Type Conversion9/1 -> Bus Creator/9  "ESP_AvhAvabliable"
  Data Type Conversion10/1 -> Bus Creator/10  "ESP_AvhStandby"
  Data Type Conversion11/1 -> Bus Creator/11  "ESP_CCSwitchOff"
  Data Type Conversion12/1 -> Bus Creator/12  "ESP_CdpActive"
  Data Type Conversion13/1 -> Bus Creator/13  "ESP_CdpAvailable"
  Data Type Conversion14/1 -> Bus Creator/14  "ESP_Driving_mode_req"
  Data Type Conversion15/1 -> Bus Creator/15  "ESP_EPBErrorStatus"
  Data Type Conversion16/1 -> Bus Creator/16  "ESP_EPBStatus"
  Data Type Conversion17/1 -> Bus Creator/17  "ESP_EPBWarningMessage1"
  Data Type Conversion18/1 -> Bus Creator/18  "ESP_EPBWarningMessage2"
  Data Type Conversion19/1 -> Bus Creator/19  "ESP_EPBWarningMessage3"
  Data Type Conversion20/1 -> Bus Creator/20  "ESP_ESPInfoLamp"
  Data Type Conversion21/1 -> Bus Creator/21  "ESP_EspCtrlActv"
  Data Type Conversion22/1 -> Bus Creator/22  "ESP_EspEnableSts"
  Data Type Conversion23/1 -> Bus Creator/23  "ESP_GearShiftPrevn"
  Data Type Conversion24/1 -> Bus Creator/24  "ESP_HBBActive_NBS"
  Data Type Conversion25/1 -> Bus Creator/25  "ESP_HBBstatus"
  Data Type Conversion26/1 -> Bus Creator/26  "ESP_HBCActive_NBS"
  Data Type Conversion27/1 -> Bus Creator/27  "ESP_HDCActive"
  Data Type Conversion28/1 -> Bus Creator/28  "ESP_HDCAvailable"
  Data Type Conversion29/1 -> Bus Creator/29  "ESP_HHCActive"
  Data Type Conversion30/1 -> Bus Creator/30  "ESP_HHCAvailable"
  Data Type Conversion31/1 -> Bus Creator/31  "ESP_LdmBLC_BLRequestController"
  Data Type Conversion32/1 -> Bus Creator/32  "ESP_SCMSts"
  Data Type Conversion33/1 -> Bus Creator/33  "ESP_TcsCtrlActv"
  Data Type Conversion34/1 -> Bus Creator/34  "ESP_TcsFlgFlt"
  Data Type Conversion35/1 -> Bus Creator/35  "ESP_VAMstatus"
  Data Type Conversion36/1 -> Bus Creator/36  "ESP_VdcFlgFlt"
  Data Type Conversion37/1 -> Bus Creator/37  "RollerBenchModeSts"
  Data Type Conversion38/1 -> Bus Creator/38  "RollingCounter_0x243"
  Bus Creator/1 -> CCAN_GW_ESP_Status_0x243FromOutData/1  "CCAN_GW_ESP_Status_0x243FromOutData"
  CCAN_GW_ESP_Status_0x243FromInData/1 -> CAN FD Unpack/1  "CCAN_GW_ESP_Status_0x243FromInData"

== system ALL_JP360_DBW_V6_5_1103/MsgFromCAN/CCAN_GW_MsgFromCAN/CCAN_GW_ESP_Tq_0x217 ==
  CCAN_GW_ESP_Tq_0x217FromInData : Inport  OutDataTypeStr=Bus:CAN_FD_MESSAGE_BUS
  Bus Creator : BusCreator  Inputs=7  OutDataTypeStr=Bus:CCAN_GW_ESP_Tq_0x217  NonVirtualBus=on
  CAN FD Unpack : canfdmsglib/CAN FD Unpack  CANdbFile=HiFire_JPT360_CCAN_Matrix_CAN_V1.72_VP_ADCU.dbc  MsgList=(none)  MsgName=ESP_Tq_0x217  ProtocolMode=CAN FD  MsgIDType=Standard (11-bit identifier)  MsgIdentifier=535  MsgLength=8  SignalInfo={'Checksum_0x217','56','8','BE','unsigned','Standard','0','1','0','0','255';'ESP_TqDecReqdByEspFast','8','16','BE','unsigned','Standard','0','0.5','-1000','-1000','1000';'ESP_TqDecReqdByEspSlow','24','16','BE','unsigned','Standard','0','0.5','-1000','-1000','1000';'ESP_TqInccReqdByEsp','40','16','BE','unsigned','Standard','0','0.5','-1000','-1000','1000';'ESP_TrqInc_Req','52','1','BE','unsigned','Standard','0','1','0','0','1';'ESP_TrqRed_Req','53','1','BE','unsigned','Standard','0','1','0','0','1';'RollingCounter_0x217','48','4','BE','unsigned','Standard','0','1','0','0','15'}  IDPort=off  TimestampPort=off  ErrorPort=off  RemotePort=off  LengthPort=off  StatusPort=off  BRSPort=off  ESIPort=off  DLCPort=off  ApplyMinMax=off
      settings: SourceProductBaseCode=XP,ME,VN  DataFormat=CANdb specified signals
  Data Type Conversion1 : DataTypeConversion  OutDataTypeStr=uint8  SaturateOnIntegerOverflow=off  RndMeth=Floor
  Data Type Conversion2 : DataTypeConversion  OutDataTypeStr=single  SaturateOnIntegerOverflow=off  RndMeth=Floor
  Data Type Conversion3 : DataTypeConversion  OutDataTypeStr=single  SaturateOnIntegerOverflow=off  RndMeth=Floor
  Data Type Conversion4 : DataTypeConversion  OutDataTypeStr=single  SaturateOnIntegerOverflow=off  RndMeth=Floor
  Data Type Conversion5 : DataTypeConversion  OutDataTypeStr=boolean  SaturateOnIntegerOverflow=off  RndMeth=Floor
  Data Type Conversion6 : DataTypeConversion  OutDataTypeStr=boolean  SaturateOnIntegerOverflow=off  RndMeth=Floor
  Data Type Conversion7 : DataTypeConversion  OutDataTypeStr=int8  SaturateOnIntegerOverflow=off  RndMeth=Floor
  CCAN_GW_ESP_Tq_0x217FromOutData : Outport  OutDataTypeStr=Bus:CCAN_GW_ESP_Tq_0x217
  wires:
  CAN FD Unpack/1 -> Data Type Conversion1/1
  CAN FD Unpack/2 -> Data Type Conversion2/1
  CAN FD Unpack/3 -> Data Type Conversion3/1
  CAN FD Unpack/4 -> Data Type Conversion4/1
  CAN FD Unpack/5 -> Data Type Conversion5/1
  CAN FD Unpack/6 -> Data Type Conversion6/1
  CAN FD Unpack/7 -> Data Type Conversion7/1
  Data Type Conversion1/1 -> Bus Creator/1  "Checksum_0x217"
  Data Type Conversion2/1 -> Bus Creator/2  "ESP_TqDecReqdByEspFast"
  Data Type Conversion3/1 -> Bus Creator/3  "ESP_TqDecReqdByEspSlow"
  Data Type Conversion4/1 -> Bus Creator/4  "ESP_TqInccReqdByEsp"
  Data Type Conversion5/1 -> Bus Creator/5  "ESP_TrqInc_Req"
  Data Type Conversion6/1 -> Bus Creator/6  "ESP_TrqRed_Req"
  Data Type Conversion7/1 -> Bus Creator/7  "RollingCounter_0x217"
  Bus Creator/1 -> CCAN_GW_ESP_Tq_0x217FromOutData/1  "CCAN_GW_ESP_Tq_0x217FromOutData"
  CCAN_GW_ESP_Tq_0x217FromInData/1 -> CAN FD Unpack/1  "CCAN_GW_ESP_Tq_0x217FromInData"
